simulink library "Navigation_Lib"  (R2014a)
settings: Solver=ode45  StartTime=0.0  StopTime=10.0  RelTol=1e-3
undefined symbols (not defined in the file or in its folder): DiscIntNeverNeededParam, gyro_x_offset, gyro_y_offset, gyro_z_offset
libraries: simulink x7, aerolibutil x5, vrlib x4, aerolibtransform2 x3, dspmtrx3 x2
(part 2 of 3)

== system Navigation_Lib/Navigation Subsystem/Attitude Determination/Calculate DCM/Update DCM ==
  Omega vector : Inport
  Gyro vector : Inport  Port=2
  "Reset_Integrator " : Inport  Port=3
  Add : Sum
  Constant : Constant  Value=0  OutDataTypeStr=double  SampleTime=1/400
  Constant1 : Constant  Commented=on  Value=0  SampleTime=-1
  Demux : Demux  Outputs=6
  Gain : Gain  Gain=-1
  Gain1 : Gain  Gain=-1
  Gain2 : Gain  Gain=-1
  Mux : Mux  Inputs=9
  Product : Product  Multiplication=Matrix(*)  RndMeth=Zero
  Reshape : Reshape  OutputDimensionality=Customize  OutputDimensions=[3,3]
  Selector1 : Selector  InputPortWidth=3  Indices=[3 2 3 1 2 1]
  Terminator : Terminator
  Unit Delay Resettable : simulink/Additional Math & Discrete/Additional Discrete/Unit Delay Resettable  vinit=eye(3,3)  tsamp=-1
  DCM Matrix : Outport  PortDimensions=[3,3]
  wires:
  Mux/1 -> Reshape/1
  Gain2/1 -> Mux/8  "-OmegaX_dt"
  Gain1/1 -> Mux/4  "-OmegaZ_dt"
  Gain/1 -> Mux/3  "-OmegaY_dt"
  Constant/1 -> Mux/9, Mux/5, Mux/1
  Demux/6 -> Gain2/1
  Demux/5 -> Mux/7  "OmegaY_dt"
  Demux/4 -> Mux/6  "OmegaX_dt"
  Demux/3 -> Gain1/1
  Demux/2 -> Gain/1
  Demux/1 -> Mux/2  "OmegaZ_dt"
  Selector1/1 -> Demux/1
  Unit Delay Resettable/1 -> Add/1, Product/1  "Previous_DCM"
  Add/1 -> DCM Matrix/1, Unit Delay Resettable/1  "DCM"
  Product/1 -> Add/2  "Temp_Matrix"
  Gyro vector/1 -> Selector1/1
  Reshape/1 -> Product/2  "Update_Matrix"
  Omega vector/1 -> Terminator/1
  "Reset_Integrator "/1 -> Unit Delay Resettable/2

== stateflow chart Navigation_Lib/Navigation Subsystem/CheckSum Pre-Processing/TempFilter/CheckSum Correction/Generate Sample Holding Pulse/Chart ==
  state Begin_State0
    entry: output =0;
  state Begin_State
    entry: output =1;
  state End_State
    entry: output=0;
  (default) -> Begin_State0
  Begin_State0 -> Begin_State : [if_transition==1]
  Begin_State -> End_State [order 1] : after(HoldDataTicks,tick)
  End_State -> Begin_State : [if_transition==1]
  Begin_State -> Begin_State [order 2] : [if_transition==1]
  data: output output; if_transition input; HoldDataTicks input

== matlab function Navigation_Lib/Navigation Subsystem/Ultrasound Estimator/Kalman Tracker ==
  data: UltraSoundMeasure input; state_correction output; covariance_correction output; covariance_correction_input input; state_correction_input input
function [state_correction, covariance_correction] = fcn(UltraSoundMeasure, covariance_correction_input,state_correction_input)


%-------------------------------
%-------------------------------
%---- Predict Stage ------------
%-------------------------------
%-------------------------------

%our states:
%  [Wx Wy Wz Bx By Bz   ]
%

p_var = 1e-2;
Ts = 1/400;
%Process Noise

Q = [p_var^2     0     
      0         p_var^2 ];

%A matrix
A =  [1   Ts    
      0   1];

%odutput these values with a unit delay (for algebraic loop), apply initial conditions
state_prediction = A*state_correction_input;
covariance_prediction_ = A*covariance_correction_input*A' + Q;

%-------------------------------
%-------------------------------
%---- Estimate Stage -----------
%-------------------------------
%-------------------------------
    %H matrix
    H = [1 0];

    %Measurement noise
    m_var = 1;
%     m_var_r = 1;

    R = [m_var^2];

    %Measurement Z
    Z = UltraSoundMeasure;

    %Compute Kalman Gain
    Kalman_Gain = covariance_prediction_*H'*inv(H*covariance_prediction_*H'+R); %2x2 matrix

    %compute state space correction based on measurement
    state_correction = state_prediction + Kalman_Gain*(Z - H*state_prediction); %2x1 vector of states

    %compute covariance correction
    covariance_correction = (eye(2) - Kalman_Gain*H)*covariance_prediction_; %2x2 covariance matrix

end

== matlab function Navigation_Lib/Navigation Subsystem/SL3D Visualization/Subsystem/Compensate 
for Magnetic Declination 
(~60 degrees in Boston)_1 ==
  data: vector_in input; y output
function y = fcn(vector_in)
%#codegen


Declination_Angle = 1*pi/3;

rot_axis = [vector_in(2) -vector_in(1)]; %find a vector perpindicular to the XY vector, such that we can pitch around it
rot_axis = rot_axis/norm(rot_axis);
%rotate by this amount
% for i=1:1:45;
% rot_angle = i*(pi/180) ;

%Define new rotation matrix
C_term = cos(Declination_Angle);
S_term = sin(Declination_Angle);
t = 1-C_term;
ux = rot_axis(1);
uy = rot_axis(2);
uz = 0; 

new_rot = [(t*ux^2 + C_term) (t*ux*uy-S_term*uz) (t*ux*uz+S_term*uy)
           (t*ux*uy+S_term*uz) (t*uy^2+C_term)     (t*uy*uz - S_term*ux)
           (t*ux*uz - S_term*uy) (t*uy*uz+S_term*ux) (t*uz^2 + C_term)];


y = new_rot*vector_in;

== system Navigation_Lib/Navigation Subsystem/Attitude Determination/Magnetometer Processing/Magnetometer Heading Calculation ==
  MagVector : Inport
  DCM : Inport  Port=2
  Compensate for Magnetic Declination (~60 degrees in Boston)_ : MATLAB Function  Commented=through  TreatAsAtomicUnit=on
  Compensate for Magnetic Declination (~67 degrees in Boston)_2 : MATLAB Function  TreatAsAtomicUnit=on
  EnlargeVectorAgain : Gain  Commented=through  Gain=3
  Transform MagVector from Body Frame to World Frame : Product  Multiplication=Matrix(*)
  Transform compensated magnetic vector into the  body frame : Product  Multiplication=Matrix(*)
  Transpose2 : dspmtrx3/Transpose  Hermitian=off  overflowFlag=off
  deg : Constant  Value=67
  Projected Mag Vector (body frame) : Outport
  Projected Mag Vector (global frame) : Outport  Port=2
  wires:
  MagVector/1 -> EnlargeVectorAgain/1
  Transform compensated magnetic vector into the  body frame/1 -> Projected Mag Vector (body frame)/1
  DCM/1 -> Transpose2/1, Transform MagVector from Body Frame to World Frame/1
  EnlargeVectorAgain/1 -> Transform MagVector from Body Frame to World Frame/2
  Transpose2/1 -> Transform compensated magnetic vector into the  body frame/1
  Transform MagVector from Body Frame to World Frame/1 -> Compensate for Magnetic Declination (~60 degrees in Boston)_/1(vector_in)
  Compensate for Magnetic Declination (~60 degrees in Boston)_/1(y) -> Compensate for Magnetic Declination (~67 degrees in Boston)_2/1(vector_in)
  Compensate for Magnetic Declination (~67 degrees in Boston)_2/1(y) -> Transform compensated magnetic vector into the  body frame/2, Projected Mag Vector (global frame)/1
  deg/1 -> Compensate for Magnetic Declination (~67 degrees in Boston)_2/2(declination_ang)

== system Navigation_Lib/Navigation Subsystem/Attitude Determination/Magnetometer Processing/Process Raw Mag Data ==
  Magnetometer : Inport
  Process Raw Mag Data (Home_330453) : Subsystem  VariantControl=TempProcessVariant==1
  Process Raw Mag Data (Work_255725) : Subsystem  VariantControl=TempProcessVariant==2
  MagVector : Outport

== system Navigation_Lib/Navigation Subsystem/Attitude Determination/Magnetometer Processing/Re-align X-axis ==
  MagVector : Inport
  Demux1 : Demux  Outputs=3
  Gain : Gain
  Gain1 : Gain  Gain=-1
  Gain2 : Gain
  Mux2 : Mux  Inputs=3
  MagVectorOut : Outport
  wires:
  Mux2/1 -> MagVectorOut/1
  Demux1/1 -> Gain1/1
  Demux1/2 -> Gain2/1
  Demux1/3 -> Gain/1
  Gain1/1 -> Mux2/1
  Gain2/1 -> Mux2/2
  Gain/1 -> Mux2/3
  MagVector/1 -> Demux1/1

== system Navigation_Lib/Navigation Subsystem/Attitude Determination/Process Accelerometer/Accelerometer Correction Offset ==
  Accelerometer : Inport
  Constant : Constant  Value=ACCEL_OFFSET_X
  Constant1 : Constant  Value=ACCEL_OFFSET_Z
  Constant2 : Constant  Value=ACCEL_OFFSET_Y
  Demux : Demux  Outputs=3
  Display : Display
  Display1 : Display
  Mux : Mux  Inputs=3
  Sum : Sum  Inputs=|++
  Sum1 : Sum  Inputs=|++
  Sum2 : Sum  Inputs=|++
  OffsetCorrection : Outport
  wires:
  Demux/1 -> Sum1/1
  Accelerometer/1 -> Display1/1, Demux/1
  Demux/3 -> Sum/1
  Sum/1 -> Mux/3
  Sum1/1 -> Mux/1
  Sum2/1 -> Mux/2
  Demux/2 -> Sum2/1
  Mux/1 -> OffsetCorrection/1, Display/1
  Constant/1 -> Sum1/2
  Constant2/1 -> Sum2/2
  Constant1/1 -> Sum/2

== system Navigation_Lib/Navigation Subsystem/Attitude Determination/Process Accelerometer/Accelerometer Neutral Gain and Offset ==
  note: All axes were invereted here, both implementations in paparazzi and student team seem to do this
  note: (1/512)g /LSB
  Raw Accel Data : Inport
  Bias : Constant  Value=[4096]
  Data Type Conversion : DataTypeConversion  OutDataTypeStr=int16
  Demux : Demux  Outputs=3
  Gain : Gain  Gain=[0.001953125, 0.001953125, 0.001953125]
  Gain1 : Gain  Gain=-1  OutDataTypeStr=double
  Gain2 : Gain  Gain=-1  OutDataTypeStr=double
  Gain3 : Gain  Gain=-1  OutDataTypeStr=double
  Mux : Mux  Inputs=3
  Neutral Bias : Constant  Value=[2048 2048 2048]
  Sum : Sum  Inputs=|++
  Sum1 : Sum  Inputs=|+-
  Sum2 : Sum  Inputs=|++
  Sum3 : Sum  Inputs=|++
  Processed Accel Data : Outport
  Accel_Pre_Norm : Outport  Port=2
  wires:
  Sum1/1 -> Gain/1
  Mux/1 -> Sum1/1
  Neutral Bias/1 -> Sum1/2
  Raw Accel Data/1 -> Data Type Conversion/1
  Demux/1 -> Gain1/1
  Sum3/1 -> Mux/1
  Demux/2 -> Gain2/1
  Gain2/1 -> Sum/1
  Sum/1 -> Mux/2
  Demux/3 -> Gain3/1
  Gain3/1 -> Sum2/1
  Sum2/1 -> Mux/3
  Bias/1 -> Sum2/2, Sum/2, Sum3/2
  Data Type Conversion/1 -> Demux/1
  Gain1/1 -> Sum3/1
  Gain/1 -> Accel_Pre_Norm/1, Processed Accel Data/1

== system Navigation_Lib/Navigation Subsystem/Attitude Determination/Process Accelerometer/Low Pass Filter ==
  Offset Accel : Inport
  Add : Sum
  Gain : Gain  Gain=0.8
  Gain1 : Gain  Gain=0.2
  Unit Delay : UnitDelay  SampleTime=-1
  Filtered Accel : Outport
  wires:
  Unit Delay/1 -> Gain/1
  Gain1/1 -> Add/1
  Gain/1 -> Add/2
  Add/1 -> Unit Delay/1, Filtered Accel/1
  Offset Accel/1 -> Gain1/1

== system Navigation_Lib/Navigation Subsystem/CheckSum Pre-Processing/Accelerometer Processing/Calculate Accel Data ==
  Raw Accel Data : Inport
  Bias : Constant  Value=[0 4096 4096]
  Gain : Gain  Gain=[0.001953125, 0.001953125, 0.001953125]
  Neutral Bias : Constant  Value=[2048 2048 2048]
  Sum : Sum  Inputs=|-+
  Sum1 : Sum  Inputs=|+-
  Processed Accel Data : Outport
  wires:
  Bias/1 -> Sum/2
  Neutral Bias/1 -> Sum1/2
  Sum/1 -> Sum1/1
  Gain/1 -> Processed Accel Data/1
  Sum1/1 -> Gain/1
  Raw Accel Data/1 -> Sum/1

== system Navigation_Lib/Navigation Subsystem/CheckSum Pre-Processing/Accelerometer Processing/CheckSum Correction ==
  CalculatedData : Inport
  CheckSumFlag : Inport  Port=2
  Holding Value : Inport  Port=3
  Compare To Zero : simulink/Logic and Bit Operations/Compare To Zero  relop=>  OutDataTypeStr=boolean
  Delay : Delay  DelayLength=3  InitialCondition=0
  Generate Sample Holding Pulse : Subsystem
  "If True, we have good data, If false, we have bad data, With bad data, use previous good data from N samples ago and hold it on that value for M samples" : Switch  Criteria=u2 > Threshold
  Invert Logic : Logic  Operator=NOT  AllPortsSameDT=off  OutDataTypeStr=boolean
  Logical Operator1 : Logic  Operator=NOT  AllPortsSameDT=off  OutDataTypeStr=boolean
  Pre-Processed Height : Outport
  wires:
  Holding Value/1 -> Generate Sample Holding Pulse/2(HoldDataTicks_Value)
  Invert Logic/1 -> "If True, we have good data, If false, we have bad data, With bad data, use previous good data from N samples ago and hold it on that value for M samples"/2
  Logical Operator1/1 -> Generate Sample Holding Pulse/1(CheckSumFlag)
  Generate Sample Holding Pulse/1(Hold_Data_Pulse) -> Invert Logic/1
  Compare To Zero/1 -> Logical Operator1/1
  Delay/1 -> "If True, we have good data, If false, we have bad data, With bad data, use previous good data from N samples ago and hold it on that value for M samples"/3
  "If True, we have good data, If false, we have bad data, With bad data, use previous good data from N samples ago and hold it on that value for M samples"/1 -> Delay/1, Pre-Processed Height/1
  CalculatedData/1 -> "If True, we have good data, If false, we have bad data, With bad data, use previous good data from N samples ago and hold it on that value for M samples"/1
  CheckSumFlag/1 -> Compare To Zero/1

== system Navigation_Lib/Navigation Subsystem/CheckSum Pre-Processing/Magnetometer/CheckSum Correction ==
  CalculatedData : Inport
  CheckSumFlag : Inport  Port=2
  Holding Value : Inport  Port=3
  Compare To Zero : simulink/Logic and Bit Operations/Compare To Zero  relop=>  OutDataTypeStr=boolean
  Delay : Delay  DelayLength=3  InitialCondition=0
  Generate Sample Holding Pulse : Subsystem
  "If True, we have good data, If false, we have bad data, With bad data, use previous good data from N samples ago and hold it on that value for M samples" : Switch  Criteria=u2 > Threshold
  Invert Logic : Logic  Operator=NOT  AllPortsSameDT=off  OutDataTypeStr=boolean
  Logical Operator1 : Logic  Operator=NOT  AllPortsSameDT=off  OutDataTypeStr=boolean
  Pre-Processed Data : Outport
  wires:
  Holding Value/1 -> Generate Sample Holding Pulse/2(HoldDataTicks_Value)
  Invert Logic/1 -> "If True, we have good data, If false, we have bad data, With bad data, use previous good data from N samples ago and hold it on that value for M samples"/2
  Logical Operator1/1 -> Generate Sample Holding Pulse/1(CheckSumFlag)
  Generate Sample Holding Pulse/1(Hold_Data_Pulse) -> Invert Logic/1
  Compare To Zero/1 -> Logical Operator1/1
  Delay/1 -> "If True, we have good data, If false, we have bad data, With bad data, use previous good data from N samples ago and hold it on that value for M samples"/3
  "If True, we have good data, If false, we have bad data, With bad data, use previous good data from N samples ago and hold it on that value for M samples"/1 -> Delay/1, Pre-Processed Data/1
  CalculatedData/1 -> "If True, we have good data, If false, we have bad data, With bad data, use previous good data from N samples ago and hold it on that value for M samples"/1
  CheckSumFlag/1 -> Compare To Zero/1

== system Navigation_Lib/Navigation Subsystem/CheckSum Pre-Processing/Magnetometer/Process Raw Mag Data ==
  note: magnetometer[ 0 ] = - ( float ) navdata.mx ;
      | magnetometer[ 1 ] = ( float ) navdata.my ;
      | magnetometer[ 2 ] = - ( float ) navdata.mz ;
      | const float Sensitivity[ 3 ] = { 0.0071492608 , 0.0070882491 , 0.0074057781 } ;
      | const float Neutral[ 3 ] = { 118.0 , - 65.0 , 110.0 } ;
  Magnetometer : Inport
  Bias : Constant  Value=[ 118.0, -65.0, 110.0 ]
  Sum : Sum  Inputs=|+-
  postGain : Gain  Gain=[0.0071492608, 0.0070882491, 0.0074057781]
  preGain : Gain  Gain=[-1 1 -1]
  ProcessedData : Outport
  wires:
  Bias/1 -> Sum/2
  preGain/1 -> Sum/1
  Sum/1 -> postGain/1
  Magnetometer/1 -> preGain/1
  postGain/1 -> ProcessedData/1

== system Navigation_Lib/Navigation Subsystem/CheckSum Pre-Processing/RateGyro Processing/CheckSum Correction ==
  CalculatedData : Inport
  CheckSumFlag : Inport  Port=2
  Holding Value : Inport  Port=3
  Compare To Zero : simulink/Logic and Bit Operations/Compare To Zero  relop=>  OutDataTypeStr=boolean
  Delay : Delay  DelayLength=3  InitialCondition=0
  Generate Sample Holding Pulse : Subsystem
  "If True, we have good data, If false, we have bad data, With bad data, use previous good data from N samples ago and hold it on that value for M samples" : Switch  Criteria=u2 > Threshold
  Invert Logic : Logic  Operator=NOT  AllPortsSameDT=off  OutDataTypeStr=boolean
  Logical Operator1 : Logic  Operator=NOT  AllPortsSameDT=off  OutDataTypeStr=boolean
  Pre-Processed Height : Outport
  wires:
  Holding Value/1 -> Generate Sample Holding Pulse/2(HoldDataTicks_Value)
  Invert Logic/1 -> "If True, we have good data, If false, we have bad data, With bad data, use previous good data from N samples ago and hold it on that value for M samples"/2
  Logical Operator1/1 -> Generate Sample Holding Pulse/1(CheckSumFlag)
  Generate Sample Holding Pulse/1(Hold_Data_Pulse) -> Invert Logic/1
  Compare To Zero/1 -> Logical Operator1/1
  Delay/1 -> "If True, we have good data, If false, we have bad data, With bad data, use previous good data from N samples ago and hold it on that value for M samples"/3
  "If True, we have good data, If false, we have bad data, With bad data, use previous good data from N samples ago and hold it on that value for M samples"/1 -> Delay/1, Pre-Processed Height/1
  CalculatedData/1 -> "If True, we have good data, If false, we have bad data, With bad data, use previous good data from N samples ago and hold it on that value for M samples"/1
  CheckSumFlag/1 -> Compare To Zero/1

== system Navigation_Lib/Navigation Subsystem/CheckSum Pre-Processing/RateGyro Processing/Process Data ==
  note: const float Sensitivity[ 3 ] = { 0.0609 , 0.0609 , 0.0609 } ;
      | const float Neutral[ 3 ] = { 0.0 , 0.0 , 0.0 } ;
      | const int16_t Offset[ 3 ] = { - 73 , 14 , - 13 } ;
      | const int16_t Noises[ 3 ] = { 35 , 35 , 15 } ;
      |
      | int16_t vRaws[ 3 ] = {
      | Navdata :: IMU :: Gyroscope :: getRawX (),
      | Navdata :: IMU :: Gyroscope :: getRawY (),
      | Navdata :: IMU :: Gyroscope :: getRawZ ()
      | } ;
      |
      | gyroscope[i] = vRaws[i] * Gyroscope :: Sensitivity[i] * M_PI / 180.0 ;
  Raw Data : Inport
  Constant : Constant  Value=[0.0, 0.0, 0.0]
  Gain : Gain  Gain=[0.0609, 0.0609, 0.0609]
  Sum : Sum  Inputs=|++
  Processed Data : Outport
  wires:
  Raw Data/1 -> Sum/1
  Constant/1 -> Sum/2
  Gain/1 -> Processed Data/1
  Sum/1 -> Gain/1

== system Navigation_Lib/Navigation Subsystem/CheckSum Pre-Processing/TempFilter/CheckSum Correction ==
  CalculatedData : Inport
  CheckSumFlag : Inport  Port=2
  Holding Value : Inport  Port=3
  Compare To Zero : simulink/Logic and Bit Operations/Compare To Zero  relop=>  OutDataTypeStr=boolean
  Delay : Delay  DelayLength=3  InitialCondition=0
  Generate Sample Holding Pulse : Subsystem
  "If True, we have good data, If false, we have bad data, With bad data, use previous good data from N samples ago and hold it on that value for M samples" : Switch  Criteria=u2 > Threshold
  Invert Logic : Logic  Operator=NOT  AllPortsSameDT=off  OutDataTypeStr=boolean
  Logical Operator1 : Logic  Operator=NOT  AllPortsSameDT=off  OutDataTypeStr=boolean
  Pre-Processed Data : Outport
  wires:
  Holding Value/1 -> Generate Sample Holding Pulse/2(HoldDataTicks_Value)
  Invert Logic/1 -> "If True, we have good data, If false, we have bad data, With bad data, use previous good data from N samples ago and hold it on that value for M samples"/2
  Logical Operator1/1 -> Generate Sample Holding Pulse/1(CheckSumFlag)
  Generate Sample Holding Pulse/1(Hold_Data_Pulse) -> Invert Logic/1
  Compare To Zero/1 -> Logical Operator1/1
  Delay/1 -> "If True, we have good data, If false, we have bad data, With bad data, use previous good data from N samples ago and hold it on that value for M samples"/3
  "If True, we have good data, If false, we have bad data, With bad data, use previous good data from N samples ago and hold it on that value for M samples"/1 -> Delay/1, Pre-Processed Data/1
  CalculatedData/1 -> "If True, we have good data, If false, we have bad data, With bad data, use previous good data from N samples ago and hold it on that value for M samples"/1
  CheckSumFlag/1 -> Compare To Zero/1

== system Navigation_Lib/Navigation Subsystem/CheckSum Pre-Processing/TempFilter/Process Raw Mag Data ==
  note: magnetometer[ 0 ] = - ( float ) navdata.mx ;
      | magnetometer[ 1 ] = ( float ) navdata.my ;
      | magnetometer[ 2 ] = - ( float ) navdata.mz ;
      | const float Sensitivity[ 3 ] = { 0.0071492608 , 0.0070882491 , 0.0074057781 } ;
      | const float Neutral[ 3 ] = { 118.0 , - 65.0 , 110.0 } ;
  Magnetometer : Inport
  Bias : Constant  Value=[ 118.0, -65.0, 110.0 ]
  Sum : Sum  Inputs=|+-
  postGain : Gain  Gain=[0.0071492608, 0.0070882491, 0.0074057781]
  preGain : Gain  Gain=[-1 1 -1]
  ProcessedData : Outport
  wires:
  Bias/1 -> Sum/2
  preGain/1 -> Sum/1
  Sum/1 -> postGain/1
  Magnetometer/1 -> preGain/1
  postGain/1 -> ProcessedData/1

== system Navigation_Lib/Navigation Subsystem/CheckSum Pre-Processing/Ultrasound Processing/CheckSum Correction ==
  CalculatedData : Inport
  CheckSumFlag : Inport  Port=2
  Holding Value : Inport  Port=3
  Compare To Zero : simulink/Logic and Bit Operations/Compare To Zero  relop=>  OutDataTypeStr=boolean
  Delay : Delay  DelayLength=3  InitialCondition=0
  Generate Sample Holding Pulse : Subsystem
  "If True, we have good data, If false, we have bad data, With bad data, use previous good data from N samples ago and hold it on that value for M samples" : Switch  Criteria=u2 > Threshold
  Invert Logic : Logic  Operator=NOT  AllPortsSameDT=off  OutDataTypeStr=boolean
  Logical Operator1 : Logic  Operator=NOT  AllPortsSameDT=off  OutDataTypeStr=boolean
  Pre-Processed Height : Outport
  wires:
  Holding Value/1 -> Generate Sample Holding Pulse/2(HoldDataTicks_Value)
  Invert Logic/1 -> "If True, we have good data, If false, we have bad data, With bad data, use previous good data from N samples ago and hold it on that value for M samples"/2
  Logical Operator1/1 -> Generate Sample Holding Pulse/1(CheckSumFlag)
  Generate Sample Holding Pulse/1(Hold_Data_Pulse) -> Invert Logic/1
  Compare To Zero/1 -> Logical Operator1/1
  Delay/1 -> "If True, we have good data, If false, we have bad data, With bad data, use previous good data from N samples ago and hold it on that value for M samples"/3
  "If True, we have good data, If false, we have bad data, With bad data, use previous good data from N samples ago and hold it on that value for M samples"/1 -> Delay/1, Pre-Processed Height/1
  CalculatedData/1 -> "If True, we have good data, If false, we have bad data, With bad data, use previous good data from N samples ago and hold it on that value for M samples"/1
  CheckSumFlag/1 -> Compare To Zero/1

== system Navigation_Lib/Navigation Subsystem/Remove Temperature Gyro Offset/TemperatureOffset (home_330453)/Convert to Celcius ==
  In1 : Inport
  Constant1 : Constant  Value=23000  OutDataTypeStr=int16
  Data Type Conversion3 : DataTypeConversion  OutDataTypeStr=int16
  Gain1 : Gain  Gain=1/280  OutDataTypeStr=double
  Sum4 : Sum  Inputs=|++
  Out1 : Outport
  wires:
  Constant1/1 -> Sum4/2
  Data Type Conversion3/1 -> Sum4/1
  In1/1 -> Data Type Conversion3/1
  Gain1/1 -> Out1/1
  Sum4/1 -> Gain1/1

== system Navigation_Lib/Navigation Subsystem/Remove Temperature Gyro Offset/TemperatureOffset (home_330453)/Temperature Correct Pitch ==
  Temp : Inport
  Constant : Constant  Value=-293.2
  Data Type Conversion : DataTypeConversion  OutDataTypeStr=int16
  Gain1 : Gain  Commented=through  Gain=0.01074
  Gain2 : Gain  Gain=0.005239
  Sum : Sum  Inputs=|++
  Offset Correct : Outport
  wires:
  Data Type Conversion/1 -> Offset Correct/1
  Temp/1 -> Gain2/1
  Gain1/1 -> Sum/1
  Sum/1 -> Data Type Conversion/1
  Constant/1 -> Sum/2
  Gain2/1 -> Gain1/1

== system Navigation_Lib/Navigation Subsystem/Remove Temperature Gyro Offset/TemperatureOffset (home_330453)/Temperature Correct Pitch1 ==
  note: % Linear model Poly2:
      | %      f(x) = p1*x^2 + p2*x + p3
      | % Coefficients (with 95% confidence bounds):
      | %        p1 =    0.006948  (0.006782, 0.007115)
      | %        p2 =       1.056  (1.041, 1.071)
      | %        p3 =      -66.21  (-66.54, -65.88)
  Temp : Inport
  Constant1 : Constant  Value=4.961
  Gain : Gain  Gain=0.009828
  Gain3 : Gain  Gain=0.4486
  Product : Product
  Sum1 : Sum  Inputs=|+++
  Offset Correct : Outport
  wires:
  Sum1/1 -> Offset Correct/1
  Constant1/1 -> Sum1/3
  Gain3/1 -> Sum1/2
  Gain/1 -> Sum1/1
  Product/1 -> Gain/1
  Temp/1 -> Product/2, Gain3/1, Product/1

== system Navigation_Lib/Navigation Subsystem/Remove Temperature Gyro Offset/TemperatureOffset (home_330453)/Temperature Correct Roll ==
  Temp : Inport
  Data Type Conversion : DataTypeConversion  OutDataTypeStr=int16
  Offset : Constant  Value=-498.8
  Slope : Gain  Gain=0.01074
  Sum : Sum  Inputs=|++
  Offset Correction : Outport
  wires:
  Temp/1 -> Slope/1
  Slope/1 -> Sum/1
  Sum/1 -> Data Type Conversion/1  "Temperature Offset Correction"
  Offset/1 -> Sum/2
  Data Type Conversion/1 -> Offset Correction/1

== system Navigation_Lib/Navigation Subsystem/Remove Temperature Gyro Offset/TemperatureOffset (home_330453)/Temperature Correct Roll1 ==
  note: f(x) = p1*x^2 + p2*x + p3
      | Coefficients (with 95% confidence bounds):
      |        p1 =     0.01851  (0.0183, 0.01872)
      |        p2 =       1.553  (1.534, 1.572)
      |        p3 =      -13.59  (-14, -13.17)
  Temp : Inport
  Constant : Constant  Commented=on  Value=-47.33
  Constant1 : Constant  Value=-72.51
  Gain : Gain  Gain=-0.004462
  Gain1 : Gain  Commented=through  Gain=0.01074
  Gain2 : Gain  Commented=through  Gain=3.139
  Gain3 : Gain  Gain=1.144
  Product : Product
  Sum : Sum  Inputs=|++
  Sum1 : Sum  Inputs=|+++
  Offset Correct : Outport
  wires:
  Sum1/1 -> Offset Correct/1
  Constant1/1 -> Sum1/3
  Gain3/1 -> Sum1/2
  Gain/1 -> Sum1/1
  Product/1 -> Gain/1
  Temp/1 -> Gain2/1
  Gain1/1 -> Sum/1
  Sum/1 -> Product/2, Gain3/1, Product/1
  Constant/1 -> Sum/2
  Gain2/1 -> Gain1/1

== system Navigation_Lib/Navigation Subsystem/Remove Temperature Gyro Offset/TemperatureOffset (home_330453)/Temperature Correct Yaw ==
  Temp : Inport
  Constant : Constant  Value=-40.65
  Data Type Conversion : DataTypeConversion  OutDataTypeStr=int16
  Gain1 : Gain  Commented=through  Gain=0.01074
  Gain2 : Gain  Gain=0.0008992
  Sum : Sum  Inputs=|++
  Offset Correct : Outport
  wires:
  Data Type Conversion/1 -> Offset Correct/1
  Temp/1 -> Gain2/1
  Gain1/1 -> Sum/1
  Sum/1 -> Data Type Conversion/1
  Constant/1 -> Sum/2
  Gain2/1 -> Gain1/1

== system Navigation_Lib/Navigation Subsystem/Remove Temperature Gyro Offset/TemperatureOffset (home_330453)/Temperature Correct Yaw1 ==
  note: f(x) = p1*x^2 + p2*x + p3
      | Coefficients (with 95% confidence bounds):
      |        p1 =    -0.00233  (-0.002509, -0.00215)
      |        p2 =        0.46  (0.444, 0.476)
      |        p3 =      -7.059  (-7.413, -6.705)
  note: f(x) = p1*x^2 + p2*x + p3
      | Coefficients (with 95% confidence bounds):
      |        p1 =     0.01851  (0.0183, 0.01872)
      |        p2 =       1.553  (1.534, 1.572)
      |        p3 =      -13.59  (-14, -13.17)
  Temp : Inport
  Constant : Constant  Commented=on  Value=-47.33
  Constant1 : Constant  Value=-7.059
  Gain : Gain  Gain=-0.00233
  Gain1 : Gain  Commented=through  Gain=0.01074
  Gain2 : Gain  Commented=through  Gain=3.139
  Gain3 : Gain  Gain=0.46
  Product : Product
  Sum : Sum  Inputs=|++
  Sum1 : Sum  Inputs=|+++
  Offset Correct : Outport
  wires:
  Sum1/1 -> Offset Correct/1
  Constant1/1 -> Sum1/3
  Gain3/1 -> Sum1/2
  Gain/1 -> Sum1/1
  Product/1 -> Gain/1
  Temp/1 -> Gain2/1
  Gain1/1 -> Sum/1
  Sum/1 -> Product/2, Gain3/1, Product/1
  Constant/1 -> Sum/2
  Gain2/1 -> Gain1/1

== system Navigation_Lib/Navigation Subsystem/Remove Temperature Gyro Offset/TemperatureOffset (work_255725)/Convert to Celcius ==
  In1 : Inport
  Constant1 : Constant  Value=23000  OutDataTypeStr=int16
  Data Type Conversion3 : DataTypeConversion  OutDataTypeStr=int16
  Gain1 : Gain  Gain=1/280  OutDataTypeStr=double
  Sum4 : Sum  Inputs=|++
  Out1 : Outport
  wires:
  Constant1/1 -> Sum4/2
  Data Type Conversion3/1 -> Sum4/1
  In1/1 -> Data Type Conversion3/1
  Gain1/1 -> Out1/1
  Sum4/1 -> Gain1/1

== system Navigation_Lib/Navigation Subsystem/Remove Temperature Gyro Offset/TemperatureOffset (work_255725)/Temperature Correct Pitch ==
  Temp : Inport
  Constant : Constant  Value=-293.2
  Data Type Conversion : DataTypeConversion  OutDataTypeStr=int16
  Gain1 : Gain  Commented=through  Gain=0.01074
  Gain2 : Gain  Gain=0.005239
  Sum : Sum  Inputs=|++
  Offset Correct : Outport
  wires:
  Data Type Conversion/1 -> Offset Correct/1
  Temp/1 -> Gain2/1
  Gain1/1 -> Sum/1
  Sum/1 -> Data Type Conversion/1
  Constant/1 -> Sum/2
  Gain2/1 -> Gain1/1

== system Navigation_Lib/Navigation Subsystem/Remove Temperature Gyro Offset/TemperatureOffset (work_255725)/Temperature Correct Pitch1 ==
  note: % Linear model Poly2:
      | %      f(x) = p1*x^2 + p2*x + p3
      | % Coefficients (with 95% confidence bounds):
      | %        p1 =    0.006948  (0.006782, 0.007115)
      | %        p2 =       1.056  (1.041, 1.071)
      | %        p3 =      -66.21  (-66.54, -65.88)
  Temp : Inport
  Constant1 : Constant  Value=-66.21
  Gain : Gain  Gain=0.006948
  Gain3 : Gain  Gain=1.056
  Product : Product
  Sum1 : Sum  Inputs=|+++
  Offset Correct : Outport
  wires:
  Sum1/1 -> Offset Correct/1
  Constant1/1 -> Sum1/3
  Gain3/1 -> Sum1/2
  Gain/1 -> Sum1/1
  Product/1 -> Gain/1
  Temp/1 -> Product/2, Gain3/1, Product/1

== system Navigation_Lib/Navigation Subsystem/Remove Temperature Gyro Offset/TemperatureOffset (work_255725)/Temperature Correct Roll ==
  Temp : Inport
  Data Type Conversion : DataTypeConversion  OutDataTypeStr=int16
  Offset : Constant  Value=-498.8
  Slope : Gain  Gain=0.01074
  Sum : Sum  Inputs=|++
  Offset Correction : Outport
  wires:
  Temp/1 -> Slope/1
  Slope/1 -> Sum/1
  Sum/1 -> Data Type Conversion/1  "Temperature Offset Correction"
  Offset/1 -> Sum/2
  Data Type Conversion/1 -> Offset Correction/1

== system Navigation_Lib/Navigation Subsystem/Remove Temperature Gyro Offset/TemperatureOffset (work_255725)/Temperature Correct Roll1 ==
  note: f(x) = p1*x^2 + p2*x + p3
      | Coefficients (with 95% confidence bounds):
      |        p1 =     0.01851  (0.0183, 0.01872)
      |        p2 =       1.553  (1.534, 1.572)
      |        p3 =      -13.59  (-14, -13.17)
  note: f(x) = p1*x^2 + p2*x + p3
      | Coefficients (with 95% confidence bounds):
      |        p1 =      0.1019  (0.068, 0.1358)
      |        p2 =      -5.199  (-7.907, -2.491)
      |        p3 =       119.8  (65.74, 173.8)
      |
      | Goodness of fit:
      |   SSE: 5.103e+04
      |   R-square: 0.7122
      |   Adjusted R-square: 0.7121
      |   RMSE: 1.13
      |
      |
      |      f(x) = p1*x^2 + p2*x + p3
      | Coefficients (with 95% confidence bounds):
      |        p1 =        1.25  (1.214, 1.287)
      |        p2 =      -125.3  (-129.1, -121.5)
      |        p3 =        3248  (3149, 3347)
  Temp : Inport
  Constant : Constant  Commented=on  Value=-47.33
  Constant1 : Constant  Value=-13.59
  Constant2 : Constant  Value=3248
  Gain : Gain  Gain=0.01851
  Gain1 : Gain  Commented=through  Gain=0.01074
  Gain2 : Gain  Commented=through  Gain=3.139
  Gain3 : Gain  Gain=1.553
  Gain4 : Gain  Gain=1.25
  Gain5 : Gain  Gain=-125.3
  Product : Product
  Product1 : Product
  Sum : Sum  Inputs=|++
  Sum1 : Sum  Inputs=|+++
  Sum2 : Sum  Inputs=|+++
  Offset Correct : Outport
  wires:
  Sum1/1 -> Offset Correct/1
  Product1/1 -> Gain4/1
  Constant2/1 -> Sum2/3
  Gain5/1 -> Sum2/2
  Gain4/1 -> Sum2/1
  Constant1/1 -> Sum1/3
  Gain3/1 -> Sum1/2
  Gain/1 -> Sum1/1
  Product/1 -> Gain/1
  Temp/1 -> Gain2/1
  Gain1/1 -> Sum/1
  Sum/1 -> Product1/2, Gain5/1, Product1/1, Gain3/1, Product/1, Product/2
  Constant/1 -> Sum/2
  Gain2/1 -> Gain1/1

== system Navigation_Lib/Navigation Subsystem/Remove Temperature Gyro Offset/TemperatureOffset (work_255725)/Temperature Correct Yaw ==
  Temp : Inport
  Constant : Constant  Value=-40.65
  Data Type Conversion : DataTypeConversion  OutDataTypeStr=int16
  Gain1 : Gain  Commented=through  Gain=0.01074
  Gain2 : Gain  Gain=0.0008992
  Sum : Sum  Inputs=|++
  Offset Correct : Outport
  wires:
  Data Type Conversion/1 -> Offset Correct/1
  Temp/1 -> Gain2/1
  Gain1/1 -> Sum/1
  Sum/1 -> Data Type Conversion/1
  Constant/1 -> Sum/2
  Gain2/1 -> Gain1/1

== system Navigation_Lib/Navigation Subsystem/Remove Temperature Gyro Offset/TemperatureOffset (work_255725)/Temperature Correct Yaw1 ==
  note: f(x) = p1*x^2 + p2*x + p3
      | Coefficients (with 95% confidence bounds):
      |        p1 =    -0.00233  (-0.002509, -0.00215)
      |        p2 =        0.46  (0.444, 0.476)
      |        p3 =      -7.059  (-7.413, -6.705)
  note: f(x) = p1*x^2 + p2*x + p3
      | Coefficients (with 95% confidence bounds):
      |        p1 =     0.01851  (0.0183, 0.01872)
      |        p2 =       1.553  (1.534, 1.572)
      |        p3 =      -13.59  (-14, -13.17)
  Temp : Inport
  Constant : Constant  Commented=on  Value=-47.33
  Constant1 : Constant  Value=-7.962
  Gain : Gain  Gain=0.009834
  Gain1 : Gain  Commented=through  Gain=0.01074
  Gain2 : Gain  Commented=through  Gain=3.139
  Gain3 : Gain  Gain=-0.4009
  Product : Product
  Sum : Sum  Inputs=|++
  Sum1 : Sum  Inputs=|+++
  Offset Correct : Outport
  wires:
  Sum1/1 -> Offset Correct/1
  Constant1/1 -> Sum1/3
  Gain3/1 -> Sum1/2
  Gain/1 -> Sum1/1
  Product/1 -> Gain/1
  Temp/1 -> Gain2/1
  Gain1/1 -> Sum/1
  Sum/1 -> Product/2, Gain3/1, Product/1
  Constant/1 -> Sum/2
  Gain2/1 -> Gain1/1

== system Navigation_Lib/Navigation Subsystem/Remove Temperature Gyro Offset/TemperatureOffset (work_255725)/Temperature Correct Yaw2 ==
  note: f(x) = p1*x^2 + p2*x + p3
      | Coefficients (with 95% confidence bounds):
      |        p1 =    -0.00233  (-0.002509, -0.00215)
      |        p2 =        0.46  (0.444, 0.476)
      |        p3 =      -7.059  (-7.413, -6.705)
  note: f(x) = p1*x^2 + p2*x + p3
      | Coefficients (with 95% confidence bounds):
      |        p1 =     0.01851  (0.0183, 0.01872)
      |        p2 =       1.553  (1.534, 1.572)
      |        p3 =      -13.59  (-14, -13.17)
  Temp : Inport
  Constant : Constant  Commented=on  Value=-47.33
  Constant1 : Constant  Value=-7.059
  Gain : Gain  Gain=-0.00233
  Gain1 : Gain  Commented=through  Gain=0.01074
  Gain2 : Gain  Commented=through  Gain=3.139
  Gain3 : Gain  Gain=0.46
  Product : Product
  Sum : Sum  Inputs=|++
  Sum1 : Sum  Inputs=|+++
  Offset Correct : Outport
  wires:
  Sum1/1 -> Offset Correct/1
  Constant1/1 -> Sum1/3
  Gain3/1 -> Sum1/2
  Gain/1 -> Sum1/1
  Product/1 -> Gain/1
  Temp/1 -> Gain2/1
  Gain1/1 -> Sum/1
  Sum/1 -> Product/2, Gain3/1, Product/1
  Constant/1 -> Sum/2
  Gain2/1 -> Gain1/1

== system Navigation_Lib/Navigation Subsystem/SL3D Visualization/Interchange Axes Mag for SL3D /Home Drone ==
  note: z
  note: x
  note: y
  note: This comes close, however, it doesnt seem that the axis changes properly
      | ie: i rotate drone, the green dot follows it. This  tells me the Z-axis is not
      |  properly placed
  In1 : Inport
  Demux1 : Demux  Outputs=3
  Gain : Gain  Gain=-1
  Gain1 : Gain
  Gain2 : Gain
  Mux2 : Mux  Inputs=3
  Out1 : Outport
  wires:
  Gain1/1 -> Mux2/1
  Demux1/2 -> Gain1/1
  Gain/1 -> Mux2/3
  Demux1/1 -> Gain/1
  Gain2/1 -> Mux2/2
  Demux1/3 -> Gain2/1
  In1/1 -> Demux1/1
  Mux2/1 -> Out1/1

== system Navigation_Lib/Navigation Subsystem/SL3D Visualization/Interchange Axes Mag for SL3D /Subsystem ==
  note: z
  note: x
  note: y
  note: This comes close, however, it doesnt seem that the axis changes properly
      | ie: i rotate drone, the green dot follows it. This  tells me the Z-axis is not
      |  properly placed
  In1 : Inport
  Demux1 : Demux  Outputs=3
  Gain : Gain
  Gain1 : Gain  Gain=-1
  Gain2 : Gain  Gain=-1
  Mux2 : Mux  Inputs=3
  Out1 : Outport
  wires:
  In1/1 -> Demux1/1
  Demux1/3 -> Gain/1
  Demux1/2 -> Gain1/1
  Mux2/1 -> Out1/1
  Gain1/1 -> Mux2/1
  Gain/1 -> Mux2/3
  Gain2/1 -> Mux2/2
  Demux1/1 -> Gain2/1

== system Navigation_Lib/Navigation Subsystem/SL3D Visualization/Interchange Axes Mag for SL3D /Work Drone ==
  note: z
  note: x
  note: y
  note: This comes close, however, it doesnt seem that the axis changes properly
      | ie: i rotate drone, the green dot follows it. This  tells me the Z-axis is not
      |  properly placed
  In1 : Inport
  Demux1 : Demux  Outputs=3
  Gain : Gain  Gain=-1
  Gain1 : Gain
  Gain2 : Gain
  Mux2 : Mux  Inputs=3
  Out1 : Outport
  wires:
  Gain1/1 -> Mux2/1
  Demux1/2 -> Gain1/1
  Gain/1 -> Mux2/3
  Demux1/1 -> Gain/1
  Gain2/1 -> Mux2/2
  Demux1/3 -> Gain2/1
  In1/1 -> Demux1/1
  Mux2/1 -> Out1/1

== system Navigation_Lib/Navigation Subsystem/SL3D Visualization/Interchange Axes Mag for SL3D /Work Drone - supposed work drone .. not really ==
  note: z
  note: x
  note: y
  note: This comes close, however, it doesnt seem that the axis changes properly
      | ie: i rotate drone, the green dot follows it. This  tells me the Z-axis is not
      |  properly placed
  In1 : Inport
  Demux1 : Demux  Outputs=3
  Gain : Gain  Gain=-1
  Gain1 : Gain
  Gain2 : Gain  Gain=-1
  Mux2 : Mux  Inputs=3
  Out1 : Outport
  wires:
  Gain1/1 -> Mux2/1
  Demux1/2 -> Gain1/1
  Gain/1 -> Mux2/3
  Demux1/1 -> Gain/1
  Gain2/1 -> Mux2/2
  Demux1/3 -> Gain2/1
  In1/1 -> Demux1/1
  Mux2/1 -> Out1/1

== system Navigation_Lib/Navigation Subsystem/Attitude Determination/Calculate DCM/Calculate Deltas/Low Pass Filter1 ==
  Input : Inport
  Delay{11..12,21..22} (4 alike) : Delay  DelayLength=1  InitialCondition=0
  SumA{21..22,31..32} (4 alike) : Sum  Inputs=|+-  RndMeth=Nearest  SaturateOnIntegerOverflow=on  OutDataTypeStr=Inherit: Same as first input
  SumB{21..22,31..32} (4 alike) : Sum  Inputs=|++  RndMeth=Nearest  SaturateOnIntegerOverflow=on  OutDataTypeStr=Inherit: Same as first input
  a(2)(1) : Gain  Gain=-1.2246464819911413  ParamDataTypeStr=double  RndMeth=Nearest  SaturateOnIntegerOverflow=on  OutDataTypeStr=Inherit: Same as input
  a(2)(2) : Gain  Gain=-1.3465055478176402  ParamDataTypeStr=double  RndMeth=Nearest  SaturateOnIntegerOverflow=on  OutDataTypeStr=Inherit: Same as input
  a(3)(1) : Gain  Gain=0.42616417218876096  ParamDataTypeStr=double  RndMeth=Nearest  SaturateOnIntegerOverflow=on  OutDataTypeStr=Inherit: Same as input
  a(3)(2) : Gain  Gain=0.77448341373041674  ParamDataTypeStr=double  RndMeth=Nearest  SaturateOnIntegerOverflow=on  OutDataTypeStr=Inherit: Same as input
  b(2)(1) : Gain  Gain=0.98859289939093931  ParamDataTypeStr=double  RndMeth=Nearest  SaturateOnIntegerOverflow=on  OutDataTypeStr=Inherit: Same as input
  b(2)(2) : Gain  Gain=-0.57608730768019933  ParamDataTypeStr=double  RndMeth=Nearest  SaturateOnIntegerOverflow=on  OutDataTypeStr=Inherit: Same as input
  s(1) : Gain  Gain=0.64277503697032301  ParamDataTypeStr=double  RndMeth=Nearest  SaturateOnIntegerOverflow=on  OutDataTypeStr=Inherit: Same as input
  s(2) : Gain  Gain=0.031169178920745725  ParamDataTypeStr=double  RndMeth=Nearest  SaturateOnIntegerOverflow=on  OutDataTypeStr=Inherit: Same as input
  Output : Outport
  wires:
  Delay22/1 -> SumB32/2, a(3)(2)/1
  a(3)(2)/1 -> SumA32/2
  b(2)(2)/1 -> SumB22/2
  Delay12/1 -> Delay22/1, b(2)(2)/1, a(2)(2)/1
  a(2)(2)/1 -> SumA22/2
  SumB32/1 -> Output/1
  SumB22/1 -> SumB32/1
  SumA32/1 -> Delay12/1, SumB22/1
  SumA22/1 -> SumA32/1
  s(2)/1 -> SumA22/1
  Delay21/1 -> SumB31/2, a(3)(1)/1
  a(3)(1)/1 -> SumA31/2
  b(2)(1)/1 -> SumB21/2
  Delay11/1 -> Delay21/1, b(2)(1)/1, a(2)(1)/1
  a(2)(1)/1 -> SumA21/2
  SumB31/1 -> s(2)/1
  SumB21/1 -> SumB31/1
  SumA31/1 -> Delay11/1, SumB21/1
  SumA21/1 -> SumA31/1
  s(1)/1 -> SumA21/1
  Input/1 -> s(1)/1

== system Navigation_Lib/Navigation Subsystem/Attitude Determination/Magnetometer Processing/Process Raw Mag Data/Process Raw Mag Data (Home_330453) ==
  note: magnetometer[ 0 ] = - ( float ) navdata.mx ;
      | magnetometer[ 1 ] = ( float ) navdata.my ;
      | magnetometer[ 2 ] = - ( float ) navdata.mz ;
      | const float Sensitivity[ 3 ] = { 0.0071492608 , 0.0070882491 , 0.0074057781 } ;
      | const float Neutral[ 3 ] = { 118.0 , - 65.0 , 110.0 } ;
  note: 158 145 136
  Magnetometer : Inport
  Bias : Constant  Value=[-23 4.3 1.44]
  Low Pass Filter1 : Subsystem  Commented=through
      mask Display: disp(['Elliptic Filter with 20 Hz corner', '\n', '44 dB stopband.'])
  Sum : Sum  Inputs=|+-
  postGain : Gain  Gain=1./[187 163 139]
  preGain : Gain  Commented=through  Gain=[1 1 1]
  MagVector : Outport
  wires:
  Low Pass Filter1/1(Output) -> MagVector/1
  Bias/1 -> Sum/2
  preGain/1 -> Sum/1
  Sum/1 -> postGain/1
  Magnetometer/1 -> preGain/1
  postGain/1 -> Low Pass Filter1/1(Input)

== system Navigation_Lib/Navigation Subsystem/Attitude Determination/Magnetometer Processing/Process Raw Mag Data/Process Raw Mag Data (Work_255725) ==
  note: magnetometer[ 0 ] = - ( float ) navdata.mx ;
      | magnetometer[ 1 ] = ( float ) navdata.my ;
      | magnetometer[ 2 ] = - ( float ) navdata.mz ;
      | const float Sensitivity[ 3 ] = { 0.0071492608 , 0.0070882491 , 0.0074057781 } ;
      | const float Neutral[ 3 ] = { 118.0 , - 65.0 , 110.0 } ;
  note: 158 145 136
  Magnetometer : Inport
  Bias : Constant  Value=[2.93 18.9 77.5]
  Low Pass Filter1 : Subsystem  Commented=through
      mask Display: disp(['Elliptic Filter with 20 Hz corner', '\n', '44 dB stopband.'])
  Sum : Sum  Inputs=|+-
  postGain : Gain  Gain=1./[167 135 132]
  preGain : Gain  Commented=through  Gain=[1 1 1]
  MagVector : Outport
  wires:
  Low Pass Filter1/1(Output) -> MagVector/1
  Bias/1 -> Sum/2
  preGain/1 -> Sum/1
  Sum/1 -> postGain/1
  Magnetometer/1 -> preGain/1
  postGain/1 -> Low Pass Filter1/1(Input)

== system Navigation_Lib/Navigation Subsystem/CheckSum Pre-Processing/Accelerometer Processing/CheckSum Correction/Generate Sample Holding Pulse ==
  CheckSumFlag : Inport
  HoldDataTicks_Value : Inport  Port=2
  Chart : Stateflow chart  TreatAsAtomicUnit=on
  Constant2 : Constant
  Logical Operator1 : Logic  AllPortsSameDT=off  OutDataTypeStr=boolean
  Transition Logic Detection : Subsystem
  Hold_Data_Pulse : Outport
  wires:
  HoldDataTicks_Value/1 -> Chart/2(HoldDataTicks)
  CheckSumFlag/1 -> Transition Logic Detection/1(Input)
  Transition Logic Detection/1(Transition Detect) -> Chart/1(if_transition)
  Chart/1(output) -> Logical Operator1/2
  Logical Operator1/1 -> Hold_Data_Pulse/1
  Constant2/1 -> Logical Operator1/1

== system Navigation_Lib/Navigation Subsystem/CheckSum Pre-Processing/Magnetometer/CheckSum Correction/Generate Sample Holding Pulse ==
  CheckSumFlag : Inport
  HoldDataTicks_Value : Inport  Port=2
  Chart : Stateflow chart  TreatAsAtomicUnit=on
  Constant2 : Constant
  Logical Operator1 : Logic  AllPortsSameDT=off  OutDataTypeStr=boolean
  Transition Logic Detection : Subsystem
  Hold_Data_Pulse : Outport
  wires:
  HoldDataTicks_Value/1 -> Chart/2(HoldDataTicks)
  CheckSumFlag/1 -> Transition Logic Detection/1(Input)
  Transition Logic Detection/1(Transition Detect) -> Chart/1(if_transition)
  Chart/1(output) -> Logical Operator1/2
  Logical Operator1/1 -> Hold_Data_Pulse/1
  Constant2/1 -> Logical Operator1/1

== system Navigation_Lib/Navigation Subsystem/CheckSum Pre-Processing/RateGyro Processing/CheckSum Correction/Generate Sample Holding Pulse ==
  CheckSumFlag : Inport
  HoldDataTicks_Value : Inport  Port=2
  Chart : Stateflow chart  TreatAsAtomicUnit=on
  Constant2 : Constant
  Logical Operator1 : Logic  AllPortsSameDT=off  OutDataTypeStr=boolean
  Transition Logic Detection : Subsystem
  Hold_Data_Pulse : Outport
  wires:
  HoldDataTicks_Value/1 -> Chart/2(HoldDataTicks)
  CheckSumFlag/1 -> Transition Logic Detection/1(Input)
  Transition Logic Detection/1(Transition Detect) -> Chart/1(if_transition)
  Chart/1(output) -> Logical Operator1/2
  Logical Operator1/1 -> Hold_Data_Pulse/1
  Constant2/1 -> Logical Operator1/1

== system Navigation_Lib/Navigation Subsystem/CheckSum Pre-Processing/TempFilter/CheckSum Correction/Generate Sample Holding Pulse ==
  CheckSumFlag : Inport
  HoldDataTicks_Value : Inport  Port=2
  Chart : Stateflow chart  TreatAsAtomicUnit=on
  Constant2 : Constant
  Logical Operator1 : Logic  AllPortsSameDT=off  OutDataTypeStr=boolean
  Transition Logic Detection : Subsystem
  Hold_Data_Pulse : Outport
  wires:
  HoldDataTicks_Value/1 -> Chart/2(HoldDataTicks)
  CheckSumFlag/1 -> Transition Logic Detection/1(Input)
  Transition Logic Detection/1(Transition Detect) -> Chart/1(if_transition)
  Chart/1(output) -> Logical Operator1/2
  Logical Operator1/1 -> Hold_Data_Pulse/1
  Constant2/1 -> Logical Operator1/1

== system Navigation_Lib/Navigation Subsystem/CheckSum Pre-Processing/Ultrasound Processing/CheckSum Correction/Generate Sample Holding Pulse ==
  CheckSumFlag : Inport
  HoldDataTicks_Value : Inport  Port=2
  Chart : Stateflow chart  TreatAsAtomicUnit=on
  Constant2 : Constant
  Logical Operator1 : Logic  AllPortsSameDT=off  OutDataTypeStr=boolean
  Transition Logic Detection : Subsystem
  Hold_Data_Pulse : Outport
  wires:
  HoldDataTicks_Value/1 -> Chart/2(HoldDataTicks)
  CheckSumFlag/1 -> Transition Logic Detection/1(Input)
  Transition Logic Detection/1(Transition Detect) -> Chart/1(if_transition)
  Chart/1(output) -> Logical Operator1/2
  Logical Operator1/1 -> Hold_Data_Pulse/1
  Constant2/1 -> Logical Operator1/1

== system Navigation_Lib/Navigation Subsystem/Attitude Determination/Magnetometer Processing/Process Raw Mag Data/Process Raw Mag Data (Home_330453)/Low Pass Filter1 ==
  Input : Inport
  Delay{11..12,21..22} (4 alike) : Delay  DelayLength=1  InitialCondition=0
  SumA{21..22,31..32} (4 alike) : Sum  Inputs=|+-  RndMeth=Nearest  SaturateOnIntegerOverflow=on  OutDataTypeStr=Inherit: Same as first input
  SumB{21..22,31..32} (4 alike) : Sum  Inputs=|++  RndMeth=Nearest  SaturateOnIntegerOverflow=on  OutDataTypeStr=Inherit: Same as first input
  a(2)(1) : Gain  Gain=-1.2246464819911413  ParamDataTypeStr=double  RndMeth=Nearest  SaturateOnIntegerOverflow=on  OutDataTypeStr=Inherit: Same as input
  a(2)(2) : Gain  Gain=-1.3465055478176402  ParamDataTypeStr=double  RndMeth=Nearest  SaturateOnIntegerOverflow=on  OutDataTypeStr=Inherit: Same as input
  a(3)(1) : Gain  Gain=0.42616417218876096  ParamDataTypeStr=double  RndMeth=Nearest  SaturateOnIntegerOverflow=on  OutDataTypeStr=Inherit: Same as input
  a(3)(2) : Gain  Gain=0.77448341373041674  ParamDataTypeStr=double  RndMeth=Nearest  SaturateOnIntegerOverflow=on  OutDataTypeStr=Inherit: Same as input
  b(2)(1) : Gain  Gain=0.98859289939093931  ParamDataTypeStr=double  RndMeth=Nearest  SaturateOnIntegerOverflow=on  OutDataTypeStr=Inherit: Same as input
  b(2)(2) : Gain  Gain=-0.57608730768019933  ParamDataTypeStr=double  RndMeth=Nearest  SaturateOnIntegerOverflow=on  OutDataTypeStr=Inherit: Same as input
  s(1) : Gain  Gain=0.64277503697032301  ParamDataTypeStr=double  RndMeth=Nearest  SaturateOnIntegerOverflow=on  OutDataTypeStr=Inherit: Same as input
  s(2) : Gain  Gain=0.031169178920745725  ParamDataTypeStr=double  RndMeth=Nearest  SaturateOnIntegerOverflow=on  OutDataTypeStr=Inherit: Same as input
  Output : Outport
  wires:
  Input/1 -> s(1)/1
  s(1)/1 -> SumA21/1
  SumA21/1 -> SumA31/1
  SumA31/1 -> SumB21/1, Delay11/1
  SumB21/1 -> SumB31/1
  SumB31/1 -> s(2)/1
  a(2)(1)/1 -> SumA21/2
  Delay11/1 -> a(2)(1)/1, b(2)(1)/1, Delay21/1
  b(2)(1)/1 -> SumB21/2
  a(3)(1)/1 -> SumA31/2
  Delay21/1 -> a(3)(1)/1, SumB31/2
  s(2)/1 -> SumA22/1
  SumA22/1 -> SumA32/1
  SumA32/1 -> SumB22/1, Delay12/1
  SumB22/1 -> SumB32/1
  SumB32/1 -> Output/1
  a(2)(2)/1 -> SumA22/2
  Delay12/1 -> a(2)(2)/1, b(2)(2)/1, Delay22/1
  b(2)(2)/1 -> SumB22/2
  a(3)(2)/1 -> SumA32/2
  Delay22/1 -> a(3)(2)/1, SumB32/2

== system Navigation_Lib/Navigation Subsystem/Attitude Determination/Magnetometer Processing/Process Raw Mag Data/Process Raw Mag Data (Work_255725)/Low Pass Filter1 ==
  Input : Inport
  Delay{11..12,21..22} (4 alike) : Delay  DelayLength=1  InitialCondition=0
  SumA{21..22,31..32} (4 alike) : Sum  Inputs=|+-  RndMeth=Nearest  SaturateOnIntegerOverflow=on  OutDataTypeStr=Inherit: Same as first input
  SumB{21..22,31..32} (4 alike) : Sum  Inputs=|++  RndMeth=Nearest  SaturateOnIntegerOverflow=on  OutDataTypeStr=Inherit: Same as first input
  a(2)(1) : Gain  Gain=-1.2246464819911413  ParamDataTypeStr=double  RndMeth=Nearest  SaturateOnIntegerOverflow=on  OutDataTypeStr=Inherit: Same as input
  a(2)(2) : Gain  Gain=-1.3465055478176402  ParamDataTypeStr=double  RndMeth=Nearest  SaturateOnIntegerOverflow=on  OutDataTypeStr=Inherit: Same as input
  a(3)(1) : Gain  Gain=0.42616417218876096  ParamDataTypeStr=double  RndMeth=Nearest  SaturateOnIntegerOverflow=on  OutDataTypeStr=Inherit: Same as input
  a(3)(2) : Gain  Gain=0.77448341373041674  ParamDataTypeStr=double  RndMeth=Nearest  SaturateOnIntegerOverflow=on  OutDataTypeStr=Inherit: Same as input
  b(2)(1) : Gain  Gain=0.98859289939093931  ParamDataTypeStr=double  RndMeth=Nearest  SaturateOnIntegerOverflow=on  OutDataTypeStr=Inherit: Same as input
  b(2)(2) : Gain  Gain=-0.57608730768019933  ParamDataTypeStr=double  RndMeth=Nearest  SaturateOnIntegerOverflow=on  OutDataTypeStr=Inherit: Same as input
  s(1) : Gain  Gain=0.64277503697032301  ParamDataTypeStr=double  RndMeth=Nearest  SaturateOnIntegerOverflow=on  OutDataTypeStr=Inherit: Same as input
  s(2) : Gain  Gain=0.031169178920745725  ParamDataTypeStr=double  RndMeth=Nearest  SaturateOnIntegerOverflow=on  OutDataTypeStr=Inherit: Same as input
  Output : Outport
  wires:
  Input/1 -> s(1)/1
  s(1)/1 -> SumA21/1
  SumA21/1 -> SumA31/1
  SumA31/1 -> SumB21/1, Delay11/1
  SumB21/1 -> SumB31/1
  SumB31/1 -> s(2)/1
  a(2)(1)/1 -> SumA21/2
  Delay11/1 -> a(2)(1)/1, b(2)(1)/1, Delay21/1
  b(2)(1)/1 -> SumB21/2
  a(3)(1)/1 -> SumA31/2
  Delay21/1 -> a(3)(1)/1, SumB31/2
  s(2)/1 -> SumA22/1
  SumA22/1 -> SumA32/1
  SumA32/1 -> SumB22/1, Delay12/1
  SumB22/1 -> SumB32/1
  SumB32/1 -> Output/1
  a(2)(2)/1 -> SumA22/2
  Delay12/1 -> a(2)(2)/1, b(2)(2)/1, Delay22/1
  b(2)(2)/1 -> SumB22/2
  a(3)(2)/1 -> SumA32/2
  Delay22/1 -> a(3)(2)/1, SumB32/2

== system Navigation_Lib/Navigation Subsystem/CheckSum Pre-Processing/Accelerometer Processing/CheckSum Correction/Generate Sample Holding Pulse/Transition Logic Detection ==
  Input : Inport
  Constant : Constant  Value=0
  Constant1 : Constant
  Logical Operator : Logic  AllPortsSameDT=off  OutDataTypeStr=boolean
  Relational Operator : RelationalOperator  Operator===  OutDataTypeStr=boolean
  Relational Operator1 : RelationalOperator  Operator===  OutDataTypeStr=boolean
  Unit Delay : UnitDelay  SampleTime=-1
  Transition Detect : Outport
  wires:
  Logical Operator/1 -> Transition Detect/1  "Transition_Detect"
  Constant1/1 -> Relational Operator1/1
  Constant/1 -> Relational Operator/2
  Relational Operator/1 -> Logical Operator/2
  Input/1 -> Unit Delay/1, Relational Operator1/2
  Unit Delay/1 -> Relational Operator/1
  Relational Operator1/1 -> Logical Operator/1
